simulink model "lo_nhiet2"  (Simulink 7.9)
settings: Solver=ode45  StartTime=0  StopTime=1000  RelTol=1e-3
libraries: simulink x1
settings Model: Creator=Vaio  LastModifiedBy=Vaio
settings DebuggingCC: SolverPrmCheckMsg=none

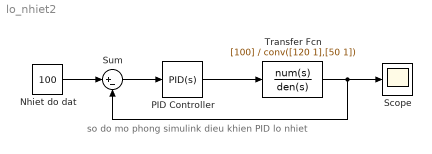
== system lo_nhiet2 ==
  note: so do mo phong simulink dieu khien PID lo nhiet
  Nhiet do dat : Constant  Value=100
  PID Controller : simulink/Continuous/PID Controller  Controller=PID  TimeDomain=Continuous-time  SampleTime=1  IntegratorMethod=Forward Euler  FilterMethod=Forward Euler  Form=Parallel  P=0.09  I=0.00225  D=0.9  N=1  InitialConditionSource=internal  InitialConditionForIntegrator=0  InitialConditionForFilter=0  ExternalReset=none  LimitOutput=off  UpperSaturationLimit=inf  LowerSaturationLimit=-inf  LinearizeAsGain=off  AntiWindupMode=none  Kb=1  TrackingMode=off  Kt=1  PParamMin=[]  PParamMax=[]  IParamMin=[]  IParamMax=[]  DParamMin=[]  DParamMax=[]  NParamMin=[]  NParamMax=[]  KbParamMin=[]  KbParamMax=[]  KtParamMin=[]  KtParamMax=[]  POutMin=[]  POutMax=[]  IOutMin=[]  IOutMax=[]  DOutMin=[]  DOutMax=[]  NOutMin=[]  NOutMax=[]  KbOutMin=[]  KbOutMax=[]  KtOutMin=[]  KtOutMax=[]  IntegratorOutMin=[]  IntegratorOutMax=[]  FilterOutMin=[]  FilterOutMax=[]  SumOutMin=[]  SumOutMax=[]  SumI1OutMin=[]  SumI1OutMax=[]  SumI2OutMin=[]  SumI2OutMax=[]  SumI3OutMin=[]  SumI3OutMax=[]  SumDOutMin=[]  SumDOutMax=[]  SaturationOutMin=[]  SaturationOutMax=[]  IntegratorContinuousStateAttributes=''  IntegratorStateMustResolveToSignalObject=off  IntegratorRTWStateStorageClass=Auto  FilterContinuousStateAttributes=''  FilterStateMustResolveToSignalObject=off  FilterRTWStateStorageClass=Auto
  Scope : Scope
  Sum : Sum  Inputs=|+-
  Transfer Fcn : TransferFcn  Numerator=[100]  Denominator=conv([120 1],[50 1])
  wires:
  PID Controller/1 -> Transfer Fcn/1
  Transfer Fcn/1 -> Scope/1, Sum/2
  Nhiet do dat/1 -> Sum/1
  Sum/1 -> PID Controller/1
